simulink model "calibration_model_feedforward"  (R2016a)
settings: Solver=FixedStepDiscrete  StartTime=0.0  StopTime=inf  FixedStep=.001  RelTol=1e-3
libraries: xpcethercatlib x7, slrtlib x4
settings Model: xpc_rtwmakecfg_data=_xpcethercatlib_  SimulationMode=external  Creator=rtheyyun  LastModifiedBy=march
settings SolverCC: EnableConcurrentExecution=on  ConcurrentTasks=on
settings DataIOCC: LimitDataPoints=on  SaveFinalState=on  SaveFormat=StructureWithTime  SignalLoggingSaveFormat=ModelDataLogs  InspectSignalLogs=on
settings OptimizationCC: BlockReduction=off  OptimizeBlockIOStorage=off  BufferReuse=off  GlobalBufferReuse=off  ExpressionFolding=off  ExpressionDepthLimit=2147483647  LocalBlockOutputs=off
settings DebuggingCC: ReadBeforeWriteMsg=DisableAll  WriteAfterWriteMsg=DisableAll  WriteAfterReadMsg=DisableAll  UnderspecifiedInitializationDetection=Classic  MergeDetectMultiDrivingBlocksExec=none  SolverPrmCheckMsg=warning  InheritedTsInSrcMsg=none  FcnCallInpInsideContextMsg=UseLocalSettings  AllowSymbolicDim=off  StateNameClashWarn=warning
settings HardwareCC: ProdBitPerPointer=32  ProdLargestAtomicFloat=None  ProdWordSize=32  ProdLongLongMode=on  ProdHWDeviceType=Generic->32-bit x86 compatible
settings ModelReferenceCC: PropagateSignalLabelsOutOfModel=off
settings RTWCC: SystemTargetFile=slrt.tlc  TemplateMakefile=slrt_default_tmf  Description=Simulink Real-Time  RTWVerbose=off  RTWCompilerOptimization=on
settings SimulinkRealTimeCC: GeneratePreprocessorConditionals=Disable all  xPCisModelTimeout=off  xPCModelTimeoutSecs=20  xPCConcurrentTasks=on
settings ConfigComp: CovModelRefEnable=Off  CovSFcnEnable=off
settings ConfigurationSet: Description=SimMechanics 2G

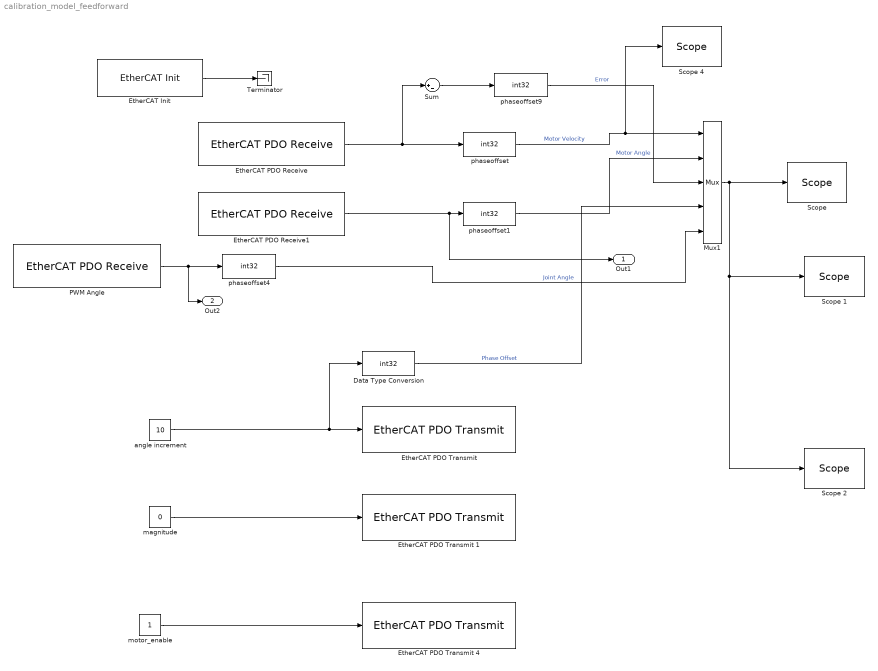
== system calibration_model_feedforward ==
  Data Type Conversion : DataTypeConversion  OutDataTypeStr=int32
  "EtherCAT Init " : xpcethercatlib/EtherCAT Init   Priority=0  config_file=D:\Software\simulink-models\EtherCAT Config files\full_setup_v1.0.xml  device_id=0  pci_bus=2  pci_slot=0  dctuning=2  enaDebug=off  enaDC=off  errLink=on  masterDbg=on  stateChgDbg=on  baseClock=off  masterCfg=on  logFile='c:\dbglog.txt'  sample_time=0.001000
  EtherCAT PDO Receive : xpcethercatlib/EtherCAT PDO Receive  Priority=2  sig_name=Right_Leg.Inputs.K_motorVelocity  sig_offset=2080  sig_type=int16  type_size=16  sig_dim=1  device_id=0  sample_time=0.001000
  EtherCAT PDO Receive1 : xpcethercatlib/EtherCAT PDO Receive  Priority=2  sig_name=Right_Leg.Inputs.K_motorAngle  sig_offset=2064  sig_type=uint16  type_size=16  sig_dim=1  device_id=0  sample_time=0.001000
  "EtherCAT PDO Transmit " : xpcethercatlib/EtherCAT PDO Transmit   Priority=3  sig_name=Right_Leg.Outputs.K_phaseOffsetNeg  sig_offset=2200  sig_type=uint16  type_size=16  sig_dim=1  device_id=0  sample_time=0.001000
  EtherCAT PDO Transmit 1 : xpcethercatlib/EtherCAT PDO Transmit   Priority=3  sig_name=Right_Leg.Outputs.K_phaseOffsetPos  sig_offset=2184  sig_type=uint16  type_size=16  sig_dim=1  device_id=0  sample_time=0.001000
  EtherCAT PDO Transmit 4 : xpcethercatlib/EtherCAT PDO Transmit   Priority=3  sig_name=Right_Leg.Outputs.K_motorEnable  sig_offset=2168  sig_type=uint8  type_size=8  sig_dim=1  device_id=0  sample_time=0.001000
  Mux1 : Mux  Inputs=5
  PWM Angle : xpcethercatlib/EtherCAT PDO Receive  Priority=2  sig_name=Right_Leg.Inputs.K_jointAngle  sig_offset=2000  sig_type=uint32  type_size=32  sig_dim=1  device_id=0  sample_time=0.001000
  "Scope " : slrtlib/Displays and Logging/Scope   scopeno=1  scopetype=Target  autostart=on  viewmode=Numerical  formatstr='%15.6f'  grid=on  ylimits=[0,0]  nosamples=3  noprepostsamples=0  interleave=1  triggermode=FreeRun  triggersignal=1  trigsignalfromport=off  triggerlevel=0.0  triggerslope=Either  triggerscope=1  triggersample=0  filename=data.dat  mode=Lazy  writesize=512  autorestart=off  dynamicfilemode=off  maxwritefilesize=512*1024^2
  Scope 1 : slrtlib/Displays and Logging/Scope   scopeno=2  scopetype=Target  autostart=on  viewmode=Graphical sliding  formatstr='%15.6f'  grid=on  ylimits=[0,0]  nosamples=5000  noprepostsamples=0  interleave=1  triggermode=FreeRun  triggersignal=1  trigsignalfromport=off  triggerlevel=0.0  triggerslope=Either  triggerscope=1  triggersample=0  filename=data.dat  mode=Lazy  writesize=512  autorestart=off  dynamicfilemode=off  maxwritefilesize=512*1024^2
  Scope 2 : slrtlib/Displays and Logging/Scope   scopeno=3  scopetype=File  autostart=on  viewmode=Graphical sliding  formatstr='%15.6f'  grid=on  ylimits=[0,0]  nosamples=50000  noprepostsamples=0  interleave=1  triggermode=FreeRun  triggersignal=1  trigsignalfromport=off  triggerlevel=0.0  triggerslope=Either  triggerscope=1  triggersample=0  filename=data.dat  mode=Lazy  writesize=512  autorestart=on  dynamicfilemode=off  maxwritefilesize=512*1024^2
  Scope 4 : slrtlib/Displays and Logging/Scope   scopeno=5  scopetype=Target  autostart=on  viewmode=Graphical rolling  formatstr='%15.6f'  grid=on  ylimits=[0,0]  nosamples=50000  noprepostsamples=0  interleave=1  triggermode=FreeRun  triggersignal=1  trigsignalfromport=off  triggerlevel=0.0  triggerslope=Either  triggerscope=1  triggersample=0  filename=data.dat  mode=Lazy  writesize=512  autorestart=off  dynamicfilemode=off  maxwritefilesize=512*1024^2
  Sum : Sum  Inputs=|+-
  Terminator : Terminator
  angle increment : Constant  Value=10  OutDataTypeStr=uint16
  magnitude : Constant  Value=0  OutDataTypeStr=uint16
  motor_enable : Constant  OutDataTypeStr=uint8
  phaseoffset{,1,4,9} (4 alike) : DataTypeConversion  OutDataTypeStr=int32
  Out1 : Outport  OutDataTypeStr=uint16
  Out2 : Outport  Port=2  OutDataTypeStr=uint32
  wires:
  Mux1/1 -> Scope 2/1, Scope 1/1, "Scope "/1
  "EtherCAT Init "/1 -> Terminator/1
  EtherCAT PDO Receive/1 -> Sum/1, phaseoffset/1
  EtherCAT PDO Receive1/1 -> Out1/1, phaseoffset1/1
  phaseoffset1/1 -> Mux1/2  "Motor Angle"
  phaseoffset/1 -> Scope 4/1, Mux1/1  "Motor Velocity"
  PWM Angle/1 -> Out2/1, phaseoffset4/1
  phaseoffset4/1 -> Mux1/5  "Joint Angle"
  phaseoffset9/1 -> Mux1/3  "Error"
  Sum/1 -> phaseoffset9/1
  angle increment/1 -> Data Type Conversion/1, "EtherCAT PDO Transmit "/1
  Data Type Conversion/1 -> Mux1/4  "Phase Offset"
  motor_enable/1 -> EtherCAT PDO Transmit 4/1
  magnitude/1 -> EtherCAT PDO Transmit 1/1
